simulink subsystem "tehrani_alv_mass_balance_v4"  (R2019b)
settings: Solver=VariableStepAuto  StartTime=0.0  StopTime=10.0  RelTol=1e-3
settings Model: Creator=RH  LastModifiedBy=RH

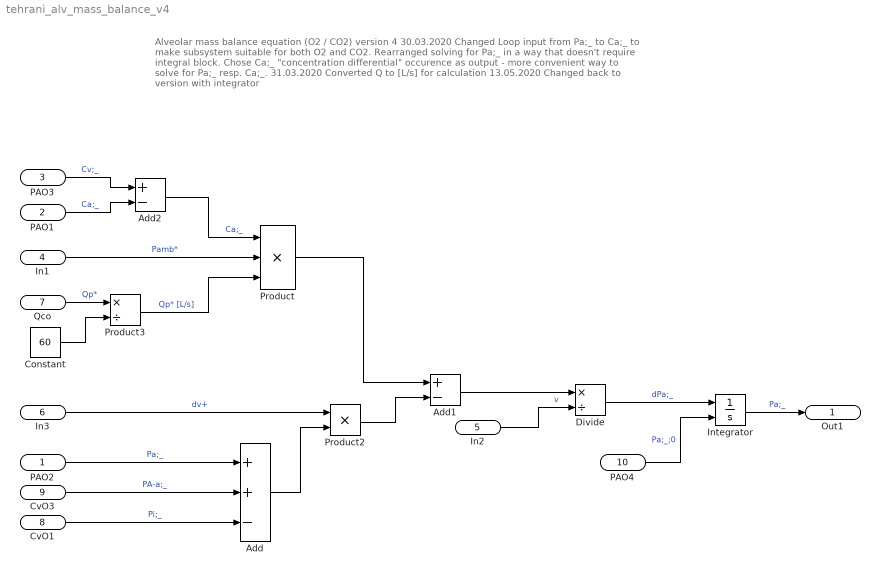
== system tehrani_alv_mass_balance_v4 ==
  note: Alveolar mass balance equation (O2 / CO2) version 4
      |
      | 30.03.2020 Changed Loop input from Pa;_ to Ca;_ to make subsystem suitable for both O2 and CO2.
      | Rearranged solving for Pa;_ in a way that doesn't require integral block.
      | Chose Ca;_ "concentration differential" occurence as output - more convenient way to solve for Pa;_ resp. Ca;_.
      | 31.03.2020 Converted Q to [L/s] for calculation
      | 13.05.2020 Changed back to version with integrator
  PAO2 : Inport  Unit=mmHg
  PAO1 : Inport  Port=2  Unit=1
  PAO3 : Inport  Port=3  Unit=1
  In1 : Inport  Port=4  Unit=mmHg
  In2 : Inport  Port=5  Unit=L
  In3 : Inport  Port=6  Unit=L/s
  Qco : Inport  Port=7  Unit=L/min
  CvO1 : Inport  Port=8  Unit=mmHg
  CvO3 : Inport  Port=9  Unit=mmHg
  PAO4 : Inport  Port=10  Unit=mmHg
  Add : Sum  Inputs=++-
  Add1 : Sum  Inputs=+-
  Add2 : Sum  Inputs=+-
  Constant : Constant  Value=60
  Divide : Product  Inputs=*/
  Integrator : Integrator  InitialConditionSource=external
  Product : Product  Inputs=***
  Product2 : Product
  Product3 : Product  Inputs=*/
  Out1 : Outport  Unit=mmHg
  wires:
  PAO4/1 -> Integrator/2  "Pa;_;0"
  Divide/1 -> Integrator/1  "dPa;_"
  Product/1 -> Add1/1
  Add2/1 -> Product/1  "Ca;_"
  PAO1/1 -> Add2/2  "Ca;_"
  Product2/1 -> Add1/2
  In2/1 -> Divide/2  "v"
  Integrator/1 -> Out1/1  "Pa;_"
  In3/1 -> Product2/1  "dv+"
  CvO1/1 -> Add/3  "Pi;_"
  PAO2/1 -> Add/1  "Pa;_"
  Qco/1 -> Product3/1  "Qp*"
  Add1/1 -> Divide/1
  In1/1 -> Product/2  "Pamb*"
  CvO3/1 -> Add/2  "PA-a;_"
  Add/1 -> Product2/2
  PAO3/1 -> Add2/1  "Cv;_"
  Product3/1 -> Product/3  "Qp* [L/s]"
  Constant/1 -> Product3/2
